simulink model "Copy_of_shake_table"  (Simulink 7.0)
settings: Solver=ode4  StartTime=0.0  StopTime=inf  FixedStep=0.001  RelTol=1e-3
undefined symbols (not defined in the file or in its folder): Den, Num, q
libraries: simulink x11, dsparch4 x5, xpclib x1
settings Model: Creator=Administrator  LastModifiedBy=msi  SimulationMode=external  BufferReuse=off
settings OptimizationCC: BlockReduction=off  OptimizeBlockIOStorage=off  BufferReuse=off  ExpressionFolding=off  LocalBlockOutputs=off
settings DebuggingCC: SaveWithParameterizedLinksMsg=none  SignalResolutionControl=TryResolveAllWithWarning
settings RTWCC: SystemTargetFile=xpctarget.tlc  TemplateMakefile=xpc_default_tmf  Description=xPC Target  ProcessScript=xpctarget_make_rtw_hook
settings xpcTargetCC: TargetFcnLib=ansi_tfl_tmw.mat  GenFloatMathFcnCalls=ANSI_C  CompOptLevelCompliant=off  PortableWordSizes=off  RL32LogBufSizeModifier=10000000

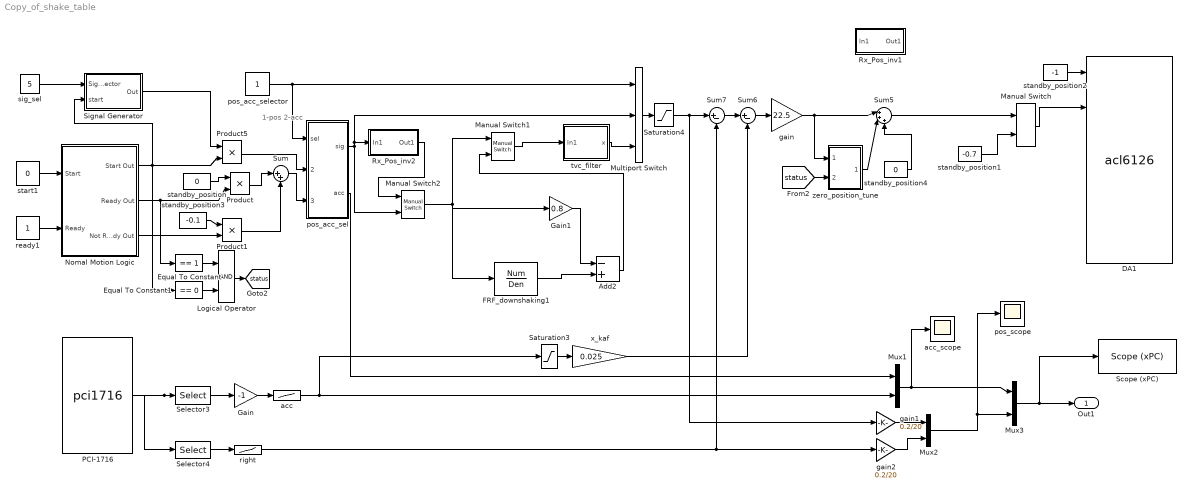
== system Copy_of_shake_table ==
  note: 1-pos
      | 2-acc
  Add2 : Sum  Inputs=-+  OutDataType=fixdt(1, 16)  OutScaling=2^-10
  DA1 : S-Function  FunctionName=acl6126  Parameters=convBaseAddr,Range,[SampleTime SampleOffset]  mask(ACL-6126){sBaseAddr=0x2C0, Ranges=-10, sample=0.001}
      mask prompts: sBaseAddr "Base Address:"; sample "Sample Time:"
      mask help:
      | ACL-6126
      | HIT
      | Analog Output
      mask init:
      | convBaseAddr = 512;Range=10;SampleTime = 0.001; SampleOffset = 0;
      | sampleLength = length (sample);
      | if (sampleLength == 2)
      |   SampleTime = sample(1);
      |   SampleOffset = sample(2);
      | else
      |   SampleTime = sample(1);
      |   SampleOffset = 0;
      | end
      | 
      | sBaseAddr(find(sBaseAddr=='''')) = [];
      | index = findstr(lower(sBaseAddr),'0x');
      | if ~isempty(index) & index==1
      |   BaseAddr = sBaseAddr(3:end);
      |   baLength = length (BaseAddr);
      |   baseStringMember = [abs('0'):abs('9'),abs('a'):abs('f'),abs('A'):abs('F')];
      |   for i = 1:baLength
      |  %   if ~ismember(BaseAddr(i),baseStringMember)
      |  %     error ('Invalid character in hexadecimal string');
      |  %   end
      |   end
      |   convBaseAddr = hex2dec(BaseAddr);
      | else
      |   convBaseAddr = str2num(BaseAddr);
      |   end
      |  Range=Ranges;
      mask Help: helpview([docroot '/toolbox/xpc/pt_io_block_reference.html#xpcioref'])
      mask Display:
      | disp('ACL-6126\ncumt\nAnalog Output');
      | port_label('input',1 , '1');
      | port_label('input',2 , '2');
      | port_label('input',3 , '3');
      | port_label('input',4 , '4');
      | port_label('input',5, '5');
      | port_label('input',6 , '6');
  Equal To Constant : simulink/Logic and Bit Operations/Compare To Constant  SystemSampleTime=-1  relop===  const=1  LogicOutDataTypeMode=uint8  ZeroCross=off
  Equal To Constant1 : simulink/Logic and Bit Operations/Compare To Constant  SystemSampleTime=-1  relop===  const=0  LogicOutDataTypeMode=uint8  ZeroCross=off
  FRF_downshaking1 : DiscreteTransferFcn  Numerator=Num  Denominator=Den  SampleTime=0.001
  Gain : Gain  Gain=-1  ParameterDataType=sfix(16)  ParameterScaling=2^0  OutDataType=sfix(16)  OutScaling=2^0  SaturateOnIntegerOverflow=on
  Gain1 : Gain  Gain=0.8  ParameterDataType=fixdt(1, 16)  ParameterScaling=2^0  OutDataType=fixdt(1, 16)  OutScaling=2^0
  Logical Operator : Logic  AllPortsSameDT=off
  Manual Switch : simulink/Signal Routing/Manual Switch  SystemSampleTime=-1  sw=1  action=0  varsize=off
  Manual Switch1 : simulink/Signal Routing/Manual Switch  SystemSampleTime=-1  sw=1  action=0  varsize=off
  Manual Switch2 : simulink/Signal Routing/Manual Switch  SystemSampleTime=-1  sw=0  action=0  varsize=off
  Multiport Switch : MultiPortSwitch  Inputs=2  SaturateOnIntegerOverflow=on
  Mux1 : Mux  Inputs=2
  Mux2 : Mux  Inputs=2
  Mux3 : Mux  Inputs=2
  Nomal Motion Logic : Subsystem  AncestorBlock=control_logic_lib/Control Logic(Stateflow Chart)
  PCI-1716 : S-Function  FunctionName=pci1716  Parameters=[SampleTime SampleOffset], SLOT  mask(hitad3){Sample=0.001, SLOT=-1}
      mask prompts: Sample "Sample Time:"
      mask help:
      | PCi1716
      | A/D Card
      | Developed by ZhaoJinsong
      | 2012.06.02
      mask init:
      | SampleTime = 0.001; SampleOffset=0;
      mask Help: helpview([docroot '/toolbox/xpc/pt_io_block_reference.html#xpcioref'])
      mask Display:
      | disp('PCI1716  ');
      | 
      | port_label('output',1 , 'OUT');
  Product : Product  OutDataType=sfix(16)  OutScaling=2^0  SaturateOnIntegerOverflow=on
  Product1 : Product  OutDataType=sfix(16)  OutScaling=2^0  SaturateOnIntegerOverflow=on
  Product5 : Product  OutDataType=sfix(16)  OutScaling=2^0  SaturateOnIntegerOverflow=on
  Rx_Pos_inv1 : Subsystem
  Rx_Pos_inv2 : Subsystem
  Saturation3 : Saturate  UpperLimit=2  LowerLimit=-2
  Saturation4 : Saturate  UpperLimit=10  LowerLimit=-10
  "Scope (xPC) " : xpclib/Misc./Scope (xPC)   SystemSampleTime=-1  scopeno=2  scopetype=Host  autostart=on  viewmode=Graphical redraw  formatstr='%15.6f'  grid=on  ylimits=[0,0]  nosamples=500  noprepostsamples=0  interleave=1  triggermode=FreeRun  triggersignal=1  triggerlevel=0.0  triggerslope=Either  triggerscope=1  triggersample=0  filename=data.dat  mode=Lazy  writesize=512  autorestart=off
  Selector3 : Selector  IndexOptions=Index vector (dialog)  Indices=[5]  OutputSizes=1
  Selector4 : Selector  IndexOptions=Index vector (dialog)  Indices=[3]  OutputSizes=1
  Signal Generator : Subsystem  TreatAsAtomicUnit=on
  Sum : Sum  Inputs=|++  OutDataType=sfix(16)  OutScaling=2^0  SaturateOnIntegerOverflow=on
  Sum5 : Sum  Inputs=|+++  OutDataType=sfix(16)  OutScaling=2^0  SaturateOnIntegerOverflow=on
  Sum6 : Sum  Inputs=|+-  OutDataType=sfix(16)  OutScaling=2^0  SaturateOnIntegerOverflow=on
  Sum7 : Sum  Inputs=|+-  OutDataType=sfix(16)  OutScaling=2^0  SaturateOnIntegerOverflow=on
  acc : Lookup  InputValues=[0.03 4.87]  Table=[0 1]  OutDataType=sfix(16)  OutScaling=2^0  SaturateOnIntegerOverflow=on
  acc_scope : Scope
      settings: TickLabels=on  TimeRange=1  YMin=-0.15  YMax=0.175
  gain : Gain  Gain=22.5  ParameterDataType=sfix(16)  ParameterScaling=2^0  OutDataType=sfix(16)  OutScaling=2^0  SaturateOnIntegerOverflow=on
  gain1 : Gain  Gain=0.2/20  ParameterDataType=sfix(16)  ParameterScaling=2^0  OutDataType=sfix(16)  OutScaling=2^0  SaturateOnIntegerOverflow=on
  gain2 : Gain  Gain=0.2/20  ParameterDataType=sfix(16)  ParameterScaling=2^0  OutDataType=sfix(16)  OutScaling=2^0  SaturateOnIntegerOverflow=on
  pos_acc_sel : Subsystem
  pos_acc_selector : Constant  OutDataType=sfix(16)  OutScaling=2^0
      settings: OpenFcn=|
      | if get_param(gcb,'value')=='1',
      | set_param(gcb,'value','2');
      | else
      | set_param(gcb,'value','1');end
  pos_scope : Scope
      settings: TickLabels=on  TimeRange=1  YMin=-0.00016  YMax=3e-005
  ready1 : Constant  OutDataType=sfix(16)  OutScaling=2^0
      settings: OpenFcn=|
      | if get_param(gcb,'value')=='1',
      | set_param(gcb,'value','0');
      | else
      | set_param(gcb,'value','1');end
  right : Lookup  InputValues=[2.007 9.834]  Table=[-10 10]  OutDataType=sfix(16)  OutScaling=2^0  SaturateOnIntegerOverflow=on
  sig_sel : Constant  Value=5  OutDataType=sfix(16)  OutScaling=2^0
  standby_position : Constant  Value=0  OutDataType=sfix(16)  OutScaling=2^0
  standby_position1 : Constant  Value=-0.7  OutDataType=sfix(16)  OutScaling=2^0
  standby_position2 : Constant  Value=-1  OutDataType=sfix(16)  OutScaling=2^0
  standby_position3 : Constant  Value=-0.1  OutDataType=sfix(16)  OutScaling=2^0
  standby_position4 : Constant  Value=0  OutDataType=sfix(16)  OutScaling=2^0
  start1 : Constant  Value=0  OutDataType=sfix(16)  OutScaling=2^0
      settings: OpenFcn=|
      | if get_param(gcb,'value')=='1',
      | set_param(gcb,'value','0');
      | else
      | set_param(gcb,'value','1');end
  tvc_filter : Subsystem
      mask Display: disp('Reference\nModule')
  x_kaf : Gain  Gain=0.025  ParameterDataType=sfix(16)  ParameterScaling=2^0  OutDataType=sfix(16)  OutScaling=2^0  SaturateOnIntegerOverflow=on
  zero_position_tune : Subsystem
  Out1 : Outport  OutDataType=sfix(16)  OutScaling=2^0
  tag scope: status=global
  wires:
  ready1/1 -> Nomal Motion Logic/2(Ready)
  start1/1 -> Nomal Motion Logic/1(Start)
  Nomal Motion Logic/2(Ready Out) -> Equal To Constant/1, Product/2
  standby_position/1 -> Product/1
  Product/1 -> Sum/1
  Sum/1 -> pos_acc_sel/3(ini_pos)
  Nomal Motion Logic/1(Start Out) -> Equal To Constant1/1, Product5/2, Signal Generator/2(start)
  Product5/1 -> pos_acc_sel/2(sig_in)
  Equal To Constant/1 -> Logical Operator/1
  Equal To Constant1/1 -> Logical Operator/2
  Logical Operator/1 -> [status]
  pos_acc_selector/1 -> Multiport Switch/1, pos_acc_sel/1(sel)
  Multiport Switch/1 -> Saturation4/1
  Saturation4/1 -> Sum7/1, gain1/1
  gain/1 -> Sum5/1, zero_position_tune/1(error_in)
  [status] -> zero_position_tune/2(status)
  zero_position_tune/1(Out) -> Sum5/2
  Sum5/1 -> Manual Switch/1
  acc/1 -> Mux1/2, Saturation3/1
  Saturation3/1 -> x_kaf/1
  x_kaf/1 -> Sum6/2
  Sum7/1 -> Sum6/1
  Sum6/1 -> gain/1
  Manual Switch/1 -> DA1/2
  gain1/1 -> Mux2/1
  PCI-1716/1 -> Selector3/1, Selector4/1
  Selector3/1 -> Gain/1
  Selector4/1 -> right/1
  Gain/1 -> acc/1
  gain2/1 -> Mux2/2
  standby_position2/1 -> DA1/1
  Mux1/1 -> Mux3/1, acc_scope/1
  Nomal Motion Logic/3(Not Ready Out) -> Product1/2
  standby_position3/1 -> Product1/1
  Mux3/1 -> "Scope (xPC) "/1, Out1/1
  Product1/1 -> Sum/2
  right/1 -> gain2/1, Sum7/2
  Mux2/1 -> Mux3/2, pos_scope/1
  standby_position1/1 -> Manual Switch/2
  sig_sel/1 -> Signal Generator/1(Signal Selector)
  Signal Generator/1(Out) -> Product5/1
  pos_acc_sel/2(acc) -> Mux1/1
  tvc_filter/1(x) -> Multiport Switch/3
  pos_acc_sel/1(sig) -> Multiport Switch/2, Rx_Pos_inv2/1(In1), Manual Switch2/2
  standby_position4/1 -> Sum5/3
  Manual Switch1/1 -> tvc_filter/1(In1)
  Gain1/1 -> Add2/1
  Add2/1 -> Manual Switch1/2
  FRF_downshaking1/1 -> Add2/2
  Manual Switch2/1 -> FRF_downshaking1/1, Manual Switch1/1, Gain1/1
  Rx_Pos_inv2/1(Out1) -> Manual Switch2/1

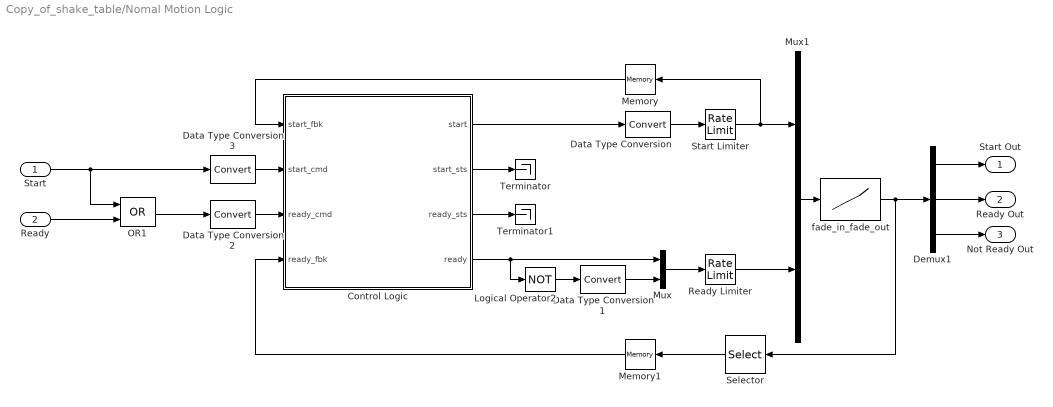
== system Copy_of_shake_table/Nomal Motion Logic ==
  Start : Inport  OutDataType=sfix(16)  OutScaling=2^0
  Ready : Inport  Port=2  OutDataType=sfix(16)  OutScaling=2^0
  Control Logic : Stateflow chart
  Data Type Conversion{,1..3} (4 alike) : DataTypeConversion  OutDataTypeMode=double  OutDataType=sfix(16)  OutScaling=2^0  SaturateOnIntegerOverflow=on  RndMeth=Zero
  Demux1 : Demux  Outputs=3
  Logical Operator2 : Logic  Operator=NOT  Inputs=3  AllPortsSameDT=off
  Memory : Memory  Orientation=left
  Memory1 : Memory  Orientation=left
  Mux : Mux  Inputs=2
  Mux1 : Mux  Inputs=2
  OR1 : Logic  Operator=OR  AllPortsSameDT=off
  Ready Limiter : RateLimiter  RisingSlewLimit=1/5  FallingSlewLimit=-1/5
  Selector : Selector  Orientation=left  InputPortWidth=3  IndexOptions=Index vector (dialog)  Indices=[2]  OutputSizes=1
  Start Limiter : RateLimiter  RisingSlewLimit=1/3  FallingSlewLimit=-1/3
  Terminator : Terminator
  Terminator1 : Terminator
  fade_in_fade_out : Lookup  InputValues=[0:0.001:1]  Table=(sin(([0:0.001:1]*2-1)*pi/2)+1)/2  OutDataType=sfix(16)  OutScaling=2^0  SaturateOnIntegerOverflow=on
  Start Out : Outport  OutDataType=sfix(16)  OutScaling=2^0
  Ready Out : Outport  Port=2  OutDataType=sfix(16)  OutScaling=2^0
  Not Ready Out : Outport  Port=3  OutDataType=sfix(16)  OutScaling=2^0
  wires:
  Ready/1 -> OR1/2
  Start/1 -> OR1/1, Data Type Conversion3/1
  Control Logic/3(ready_sts) -> Terminator1/1
  Control Logic/2(start_sts) -> Terminator/1
  OR1/1 -> Data Type Conversion2/1
  Data Type Conversion3/1 -> Control Logic/2(start_cmd)
  Demux1/3 -> Not Ready Out/1
  Demux1/1 -> Start Out/1
  Demux1/2 -> Ready Out/1
  Data Type Conversion/1 -> Start Limiter/1
  Start Limiter/1 -> Mux1/1, Memory/1
  Control Logic/1(start) -> Data Type Conversion/1
  Control Logic/4(ready) -> Logical Operator2/1, Mux/1
  Logical Operator2/1 -> Data Type Conversion1/1
  Mux/1 -> Ready Limiter/1
  Ready Limiter/1 -> Mux1/2
  Mux1/1 -> fade_in_fade_out/1
  fade_in_fade_out/1 -> Selector/1, Demux1/1
  Memory/1 -> Control Logic/1(start_fbk)
  Memory1/1 -> Control Logic/4(ready_fbk)
  Data Type Conversion1/1 -> Mux/2
  Data Type Conversion2/1 -> Control Logic/3(ready_cmd)
  Selector/1 -> Memory1/1

== system Copy_of_shake_table/Rx_Pos_inv1 ==
  In1 : Inport  OutDataType=sfix(16)  OutScaling=2^0
  Discrete Transfer Fcn1 : DiscreteTransferFcn  Numerator=[1 -0.2361]  Denominator=[1 0.3425]  SampleTime=0.001
  Discrete Transfer Fcn2 : DiscreteTransferFcn  Numerator=[1 -1.404 0.4961]  Denominator=[1 -1.59 0.7902]  SampleTime=0.001
  Discrete Transfer Fcn3 : DiscreteTransferFcn  Numerator=[1 -1.808 0.9141]  Denominator=[1.666 -2.372 1]  SampleTime=0.001
  Discrete Transfer Fcn4 : DiscreteTransferFcn  Numerator=[1 1.076 0.8841]  Denominator=[1 -1.303 0.8939]  SampleTime=0.001
  Discrete Transfer Fcn6 : DiscreteTransferFcn  Numerator=[1 -0.06054 0.6042]  Denominator=[1 0.5145 0.7374]  SampleTime=0.001
  Gain : Gain  Gain=1/0.31645  ParameterDataType=sfix(16)  ParameterScaling=2^0  OutDataType=sfix(16)  OutScaling=2^0
  Gain1 : Gain  ParameterDataType=sfix(16)  ParameterScaling=2^0  OutDataType=sfix(16)  OutScaling=2^0
  Out1 : Outport  OutDataType=sfix(16)  OutScaling=2^0
  wires:
  Discrete Transfer Fcn1/1 -> Discrete Transfer Fcn2/1
  Discrete Transfer Fcn2/1 -> Discrete Transfer Fcn3/1
  Discrete Transfer Fcn3/1 -> Discrete Transfer Fcn4/1
  Discrete Transfer Fcn4/1 -> Discrete Transfer Fcn6/1
  Discrete Transfer Fcn6/1 -> Gain/1
  In1/1 -> Discrete Transfer Fcn1/1
  Gain/1 -> Gain1/1
  Gain1/1 -> Out1/1

== system Copy_of_shake_table/Rx_Pos_inv2 ==
  In1 : Inport  OutDataType=sfix(16)  OutScaling=2^0
  Discrete Transfer Fcn1 : DiscreteTransferFcn  Numerator=[1 0.2074]  Denominator=[1.002 -1]  SampleTime=0.001
  Discrete Transfer Fcn2 : DiscreteTransferFcn  Numerator=[1 -1]  Denominator=[1 -0.8636]  SampleTime=0.001
  Discrete Transfer Fcn3 : DiscreteTransferFcn  Numerator=[1 -1.866 0.8774]  Denominator=[1 -1.762 0.9049]  SampleTime=0.001
  Discrete Transfer Fcn4 : DiscreteTransferFcn  Numerator=[1 -1.828 0.9273]  Denominator=[1 -0.4559 0.3103]  SampleTime=0.001
  Discrete Transfer Fcn5 : DiscreteTransferFcn  Numerator=[1 -1.652 0.9951]  Denominator=[1.96 -2.518 1]  SampleTime=0.001
  Discrete Transfer Fcn6 : DiscreteTransferFcn  Numerator=[1 -1.779 0.9237]  Denominator=[1 -1.656 0.9996]  SampleTime=0.001
  Gain : Gain  Gain=1/0.02213  ParameterDataType=sfix(16)  ParameterScaling=2^0  OutDataType=sfix(16)  OutScaling=2^0
  Gain1 : Gain  ParameterDataType=sfix(16)  ParameterScaling=2^0  OutDataType=sfix(16)  OutScaling=2^0
  Out1 : Outport  OutDataType=sfix(16)  OutScaling=2^0
  wires:
  Discrete Transfer Fcn1/1 -> Discrete Transfer Fcn2/1
  Discrete Transfer Fcn2/1 -> Discrete Transfer Fcn3/1
  Discrete Transfer Fcn3/1 -> Discrete Transfer Fcn4/1
  Discrete Transfer Fcn4/1 -> Discrete Transfer Fcn6/1
  Discrete Transfer Fcn6/1 -> Discrete Transfer Fcn5/1
  In1/1 -> Discrete Transfer Fcn1/1
  Gain/1 -> Gain1/1
  Gain1/1 -> Out1/1
  Discrete Transfer Fcn5/1 -> Gain/1

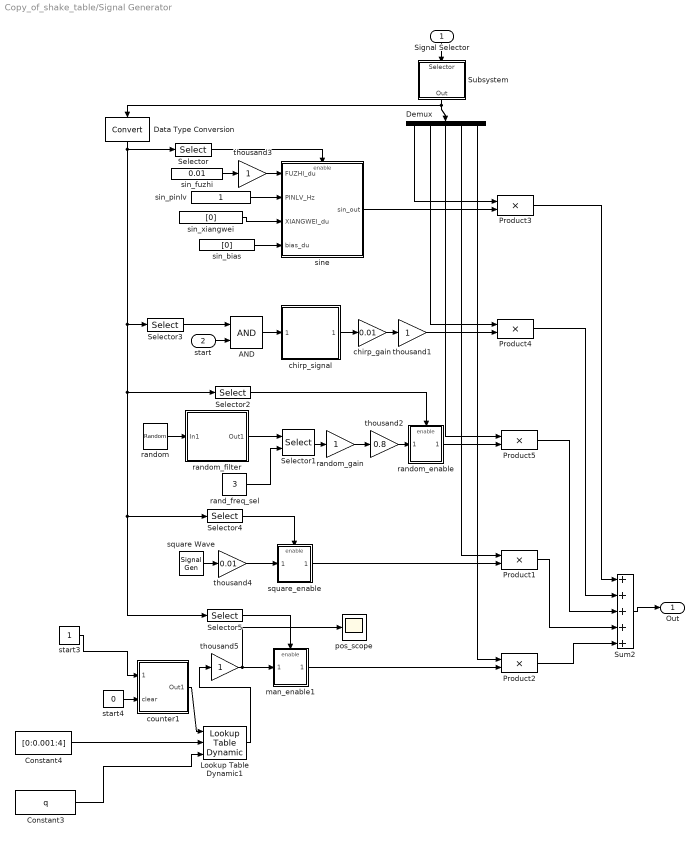
== system Copy_of_shake_table/Signal Generator ==
  Signal Selector : Inport  Orientation=down  OutDataType=sfix(16)  OutScaling=2^0
  start : Inport  Port=2  OutDataType=sfix(16)  OutScaling=2^0
  AND : Logic  AllPortsSameDT=off  OutDataTypeMode=Specify via dialog
  Constant3 : Constant  Value=q  OutDataType=sfix(16)  OutScaling=2^0
  Constant4 : Constant  Value=[0:0.001:4]  OutDataType=sfix(16)  OutScaling=2^0
  Data Type Conversion : DataTypeConversion  Orientation=down  OutDataTypeMode=boolean  OutDataType=sfix(16)  OutScaling=2^0  SaturateOnIntegerOverflow=on  RndMeth=Zero
  Demux : Demux  Orientation=down  Outputs=5
  Lookup Table Dynamic1 : simulink/Lookup Tables/Lookup Table Dynamic  LookUpMeth=Interpolation-Use End Values  OutDataTypeStr=float('double')  OutputDataTypeScalingMode=Specify via dialog  OutDataType=float('double')  OutScaling=2^-10  DoSatur=off
  Product{1..5} (5 alike) : Product  OutDataType=sfix(16)  OutScaling=2^0  SaturateOnIntegerOverflow=on
  Selector : Selector  InputPortWidth=5  IndexOptions=Index vector (dialog)  Indices=1  OutputSizes=1
  Selector1 : Selector  InputPortWidth=5  IndexOptions=Index vector (port)  Indices=[1 3]  OutputSizes=1
  Selector2 : Selector  InputPortWidth=5  IndexOptions=Index vector (dialog)  Indices=3  OutputSizes=1
  Selector3 : Selector  InputPortWidth=5  IndexOptions=Index vector (dialog)  Indices=2  OutputSizes=1
  Selector4 : Selector  InputPortWidth=5  IndexOptions=Index vector (dialog)  Indices=4  OutputSizes=1
  Selector5 : Selector  InputPortWidth=5  IndexOptions=Index vector (dialog)  Indices=5  OutputSizes=1
  Subsystem : Subsystem  Orientation=down  mask{itnum=5}
      mask prompts: itnum "Signals Number"
  Sum2 : Sum  Inputs=+++++  OutDataType=sfix(16)  OutScaling=2^0  SaturateOnIntegerOverflow=on
  chirp_gain : Gain  Gain=0.01  ParameterDataType=sfix(16)  ParameterScaling=2^0  OutDataType=sfix(16)  OutScaling=2^0  SaturateOnIntegerOverflow=on
  chirp_signal : Subsystem
  counter1 : Subsystem
  man_enable1 : Subsystem  TreatAsAtomicUnit=on
  pos_scope : Scope
      settings: TickLabels=on  TimeRange=1  YMin=-4.25  YMax=0.75  SaveName=ScopeData2
  rand_freq_sel : Constant  Value=3  OutDataType=sfix(16)  OutScaling=2^0
  random : UniformRandomNumber  SampleTime=0
  random_enable : Subsystem  TreatAsAtomicUnit=on
  random_filter : Subsystem
  random_gain : Gain  ParameterDataType=sfix(16)  ParameterScaling=2^0  OutDataType=sfix(16)  OutScaling=2^0  SaturateOnIntegerOverflow=on
  sin_bias : Constant  Value=[0]  OutDataType=sfix(16)  OutScaling=2^0
  sin_fuzhi : Constant  Value=0.01  OutDataType=sfix(16)  OutScaling=2^0
  sin_pinlv : Constant  OutDataType=sfix(16)  OutScaling=2^0
  sin_xiangwei : Constant  Value=[0]  OutDataType=sfix(16)  OutScaling=2^0
  sine : Subsystem
  square Wave : SignalGenerator  WaveForm=square  Frequency=0.1
  square_enable : Subsystem  TreatAsAtomicUnit=on
  start3 : Constant  OutDataType=sfix(16)  OutScaling=2^0
      settings: OpenFcn=|
      | if strcmp(get_param(gcb,'Value'),'1')
      | set_param(gcb,'Value','0');
      | else
      | set_param(gcb,'Value','1');
      | end;
  start4 : Constant  Value=0  OutDataType=sfix(16)  OutScaling=2^0
      settings: OpenFcn=|
      | if strcmp(get_param(gcb,'Value'),'1')
      | set_param(gcb,'Value','0');
      | else
      | set_param(gcb,'Value','1');
      | end;
  thousand1 : Gain  ParameterDataType=sfix(16)  ParameterScaling=2^0  OutDataType=sfix(16)  OutScaling=2^0  SaturateOnIntegerOverflow=on
  thousand2 : Gain  Gain=0.8  ParameterDataType=sfix(16)  ParameterScaling=2^0  OutDataType=sfix(16)  OutScaling=2^0  SaturateOnIntegerOverflow=on
  thousand3 : Gain  ParameterDataType=sfix(16)  ParameterScaling=2^0  OutDataType=sfix(16)  OutScaling=2^0  SaturateOnIntegerOverflow=on
  thousand4 : Gain  Gain=0.01  ParameterDataType=sfix(16)  ParameterScaling=2^0  OutDataType=sfix(16)  OutScaling=2^0  SaturateOnIntegerOverflow=on
  thousand5 : Gain  ParameterDataType=sfix(16)  ParameterScaling=2^0  OutDataType=sfix(16)  OutScaling=2^0  SaturateOnIntegerOverflow=on
  Out : Outport  OutDataType=sfix(16)  OutScaling=2^0
  wires:
  thousand1/1 -> Product4/2
  chirp_signal/1(chirp_signal) -> chirp_gain/1
  AND/1 -> chirp_signal/1(enable)
  chirp_gain/1 -> thousand1/1
  start/1 -> AND/2
  Selector3/1 -> AND/1
  thousand4/1 -> square_enable/1(In1)
  thousand3/1 -> sine/1(FUZHI_du)
  square_enable/1(Out1) -> Product1/2
  Selector4/1 -> square_enable/Enable
  square Wave/1 -> thousand4/1
  random_gain/1 -> thousand2/1
  thousand2/1 -> random_enable/1(In1)
  Selector1/1 -> random_gain/1
  Signal Selector/1 -> Subsystem/1(Selector)
  Product4/1 -> Sum2/2
  Product3/1 -> Sum2/1
  Product5/1 -> Sum2/3
  Sum2/1 -> Out/1
  Subsystem/1(Out) -> Demux/1, Data Type Conversion/1
  sin_bias/1 -> sine/4(bias_du)
  sin_xiangwei/1 -> sine/3(XIANGWEI_du)
  sin_pinlv/1 -> sine/2(PINLV_Hz)
  sin_fuzhi/1 -> thousand3/1
  Selector/1 -> sine/Enable
  Data Type Conversion/1 -> Selector/1, Selector3/1, Selector2/1, Selector4/1, Selector5/1
  random/1 -> random_filter/1(In1)
  random_filter/1(Out1) -> Selector1/1
  rand_freq_sel/1 -> Selector1/2
  Selector2/1 -> random_enable/Enable
  Demux/1 -> Product3/1
  sine/1(sin_out) -> Product3/2
  Demux/2 -> Product4/1
  Demux/3 -> Product5/1
  random_enable/1(Out1) -> Product5/2
  Demux/4 -> Product1/1
  Product1/1 -> Sum2/4
  Selector5/1 -> man_enable1/Enable
  man_enable1/1(Out1) -> Product2/2
  Demux/5 -> Product2/1
  Product2/1 -> Sum2/5
  thousand5/1 -> man_enable1/1(In1), pos_scope/1
  Constant4/1 -> Lookup Table Dynamic1/2
  Constant3/1 -> Lookup Table Dynamic1/3
  start3/1 -> counter1/1(codition)
  start4/1 -> counter1/2(clear)
  counter1/1(Out1) -> Lookup Table Dynamic1/1
  Lookup Table Dynamic1/1 -> thousand5/1

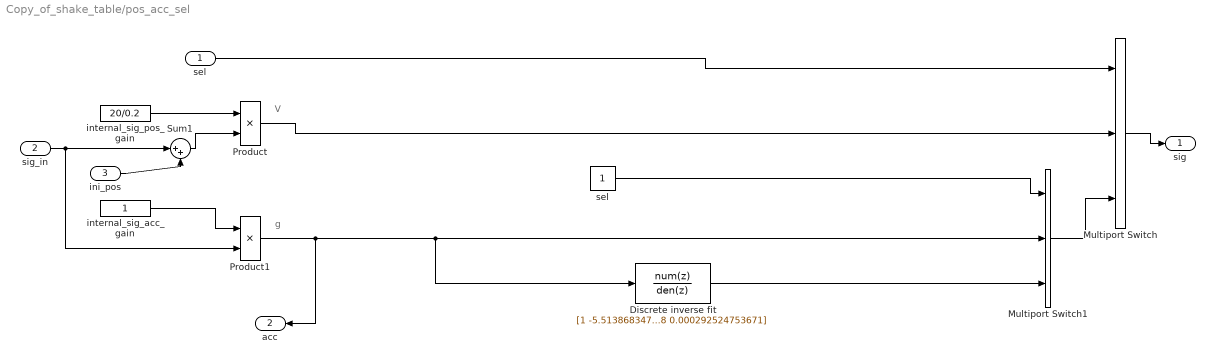
== system Copy_of_shake_table/pos_acc_sel ==
  note: g
  note: V
  sel : Inport  OutDataType=sfix(16)  OutScaling=2^0
  sig_in : Inport  Port=2  OutDataType=sfix(16)  OutScaling=2^0
  ini_pos : Inport  Port=3  OutDataType=sfix(16)  OutScaling=2^0
  Discrete inverse fit : DiscreteTransferFcn  Numerator=[1 -5.513868347662695 12.88491366007906 -16.323990002559352 11.821537968329908 -4.639485908156727 0.77101716333547]  Denominator=[0.013392688630559 -0.043519228995354 0.057088791124972 -0.038794303856191 0.015270049598488 -0.003637012524308 0.000292524753671]  SampleTime=0.001
  Multiport Switch : MultiPortSwitch  Inputs=2  SaturateOnIntegerOverflow=on
  Multiport Switch1 : MultiPortSwitch  Inputs=2  SaturateOnIntegerOverflow=on
  Product : Product  OutDataType=sfix(16)  OutScaling=2^0  SaturateOnIntegerOverflow=on
  Product1 : Product  OutDataType=sfix(16)  OutScaling=2^0  SaturateOnIntegerOverflow=on
  Sum1 : Sum  Inputs=|++  OutDataType=sfix(16)  OutScaling=2^0  SaturateOnIntegerOverflow=on
  internal_sig_acc_gain : Constant  OutDataType=sfix(16)  OutScaling=2^0
  internal_sig_pos_gain : Constant  Value=20/0.2  OutDataType=sfix(16)  OutScaling=2^0
  "sel " : Constant  OutDataType=sfix(16)  OutScaling=2^0
  sig : Outport  OutDataType=sfix(16)  OutScaling=2^0
  acc : Outport  Orientation=left  Port=2  OutDataType=sfix(16)  OutScaling=2^0
  wires:
  internal_sig_acc_gain/1 -> Product1/1
  Product1/1 -> Discrete inverse fit/1, Multiport Switch1/2, acc/1
  internal_sig_pos_gain/1 -> Product/1
  Product/1 -> Multiport Switch/2
  Sum1/1 -> Product/2
  ini_pos/1 -> Sum1/2
  Multiport Switch/1 -> sig/1
  sel/1 -> Multiport Switch/1
  sig_in/1 -> Product1/2, Sum1/1
  Discrete inverse fit/1 -> Multiport Switch1/3
  "sel "/1 -> Multiport Switch1/1
  Multiport Switch1/1 -> Multiport Switch/3

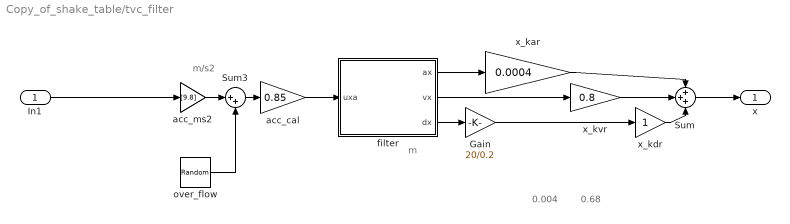
== system Copy_of_shake_table/tvc_filter ==
  note: m/s2
  note: m
  note: 0.004
  note: 0.68
  In1 : Inport  OutDataType=sfix(16)  OutScaling=2^0
  Gain : Gain  Gain=20/0.2  ParameterDataType=sfix(16)  ParameterScaling=2^0  OutDataType=sfix(16)  OutScaling=2^0  SaturateOnIntegerOverflow=on
  Sum : Sum  Inputs=+++  OutDataType=sfix(16)  OutScaling=2^0  SaturateOnIntegerOverflow=on
  Sum3 : Sum  Inputs=|++  OutDataType=sfix(16)  OutScaling=2^0  SaturateOnIntegerOverflow=on
  acc_cal : Gain  Gain=0.85  ParameterDataType=sfix(16)  ParameterScaling=2^0  OutDataType=sfix(16)  OutScaling=2^0  SaturateOnIntegerOverflow=on
  acc_ms2 : Gain  Gain=[9.8]  ParameterDataType=sfix(16)  ParameterScaling=2^0  OutDataType=sfix(16)  OutScaling=2^0  SaturateOnIntegerOverflow=on
  filter : Subsystem
      mask Display: disp('x_filter')
  over_flow : RandomNumber  Variance=1e-10  SampleTime=0
  x_kar : Gain  Gain=0.0004  ParameterDataType=sfix(16)  ParameterScaling=2^0  OutDataType=sfix(16)  OutScaling=2^0  SaturateOnIntegerOverflow=on
  x_kdr : Gain  ParameterDataType=sfix(16)  ParameterScaling=2^0  OutDataType=sfix(16)  OutScaling=2^0  SaturateOnIntegerOverflow=on
  x_kvr : Gain  Gain=0.8  ParameterDataType=sfix(16)  ParameterScaling=2^0  OutDataType=sfix(16)  OutScaling=2^0  SaturateOnIntegerOverflow=on
  x : Outport  OutDataType=sfix(16)  OutScaling=2^0
  wires:
  over_flow/1 -> Sum3/2
  In1/1 -> acc_ms2/1
  Sum3/1 -> acc_cal/1
  acc_ms2/1 -> Sum3/1
  acc_cal/1 -> filter/1(uxa)
  x_kdr/1 -> Sum/3
  x_kvr/1 -> Sum/2
  x_kar/1 -> Sum/1
  filter/1(ax) -> x_kar/1
  filter/2(vx) -> x_kvr/1
  filter/3(dx) -> Gain/1
  Sum/1 -> x/1
  Gain/1 -> x_kdr/1

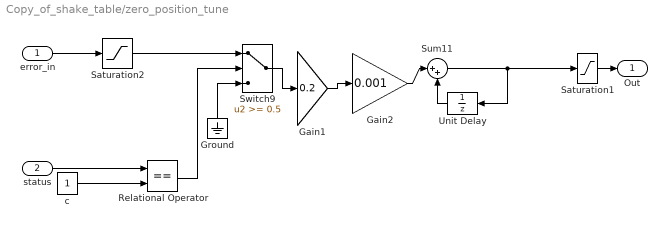
== system Copy_of_shake_table/zero_position_tune ==
  error_in : Inport  OutDataType=sfix(16)  OutScaling=2^0
  status : Inport  Port=2  OutDataType=sfix(16)  OutScaling=2^0
  Gain1 : Gain  Gain=0.2  ParameterDataType=sfix(16)  ParameterScaling=2^0  OutDataType=sfix(16)  OutScaling=2^0  SaturateOnIntegerOverflow=on
  Gain2 : Gain  Gain=0.001  ParameterDataType=sfix(16)  ParameterScaling=2^0  OutDataType=sfix(16)  OutScaling=2^0  SaturateOnIntegerOverflow=on
  Ground : Ground  Orientation=up
  Relational Operator : RelationalOperator  Operator===  InputSameDT=on
  Saturation1 : Saturate
  Saturation2 : Saturate  UpperLimit=0.1  LowerLimit=-0.1
  Sum11 : Sum  Inputs=|++  OutDataType=sfix(16)  OutScaling=2^0  SaturateOnIntegerOverflow=on  InputSameDT=on
  Switch9 : Switch  Threshold=0.5  SaturateOnIntegerOverflow=on  InputSameDT=on
  Unit Delay : UnitDelay  Orientation=left  X0=-0.03  SampleTime=0.001
  c : Constant  OutDataTypeMode=boolean  OutDataType=sfix(16)  OutScaling=2^0
  Out : Outport  OutDataType=sfix(16)  OutScaling=2^0
  wires:
  Saturation1/1 -> Out/1
  Gain1/1 -> Gain2/1
  status/1 -> Relational Operator/1
  error_in/1 -> Saturation2/1
  Relational Operator/1 -> Switch9/2
  c/1 -> Relational Operator/2
  Saturation2/1 -> Switch9/1
  Ground/1 -> Switch9/3
  Switch9/1 -> Gain1/1
  Sum11/1 -> Saturation1/1, Unit Delay/1
  Gain2/1 -> Sum11/1
  Unit Delay/1 -> Sum11/2

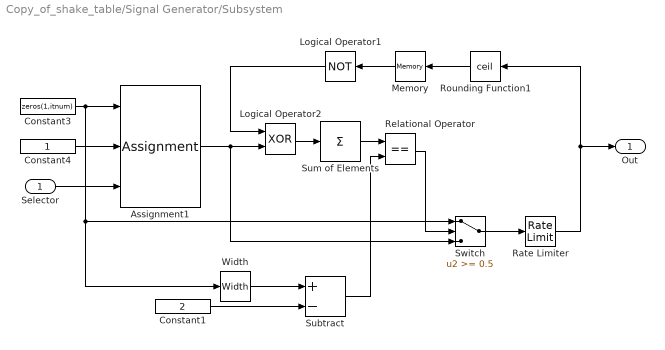
== system Copy_of_shake_table/Signal Generator/Subsystem ==
  Selector : Inport  OutDataType=sfix(16)  OutScaling=2^0
  Assignment1 : Assignment  IndexOptions=Index vector (port)  Indices=1  OutputSizes=[1]
  Constant1 : Constant  Value=2  OutDataType=sfix(16)  OutScaling=2^0
  Constant3 : Constant  Value=zeros(1,itnum)  OutDataType=sfix(16)  OutScaling=2^0
  Constant4 : Constant  OutDataType=sfix(16)  OutScaling=2^0
  Logical Operator1 : Logic  Orientation=left  Operator=NOT  AllPortsSameDT=off
  Logical Operator2 : Logic  Operator=XOR  AllPortsSameDT=off
  Memory : Memory  Orientation=left  InheritSampleTime=on
  Rate Limiter : RateLimiter
  Relational Operator : RelationalOperator  Operator===
  Rounding Function1 : Rounding  Orientation=left  Operator=ceil
  Subtract : Sum  Inputs=+-  OutDataTypeMode=double  OutDataType=sfix(16)  OutScaling=2^-10
  Sum of Elements : Sum  Inputs=+  OutDataTypeMode=double  OutDataType=sfix(16)  OutScaling=2^-10
  Switch : Switch  Threshold=0.5  SaturateOnIntegerOverflow=on
  Width : Width
  Out : Outport  OutDataType=sfix(16)  OutScaling=2^0
  wires:
  Constant3/1 -> Assignment1/1, Width/1, Switch/1
  Constant4/1 -> Assignment1/2
  Assignment1/1 -> Logical Operator2/2, Switch/3
  Rate Limiter/1 -> Rounding Function1/1, Out/1
  Rounding Function1/1 -> Memory/1
  Logical Operator1/1 -> Logical Operator2/1
  Switch/1 -> Rate Limiter/1
  Memory/1 -> Logical Operator1/1
  Selector/1 -> Assignment1/3
  Logical Operator2/1 -> Sum of Elements/1
  Width/1 -> Subtract/1
  Constant1/1 -> Subtract/2
  Sum of Elements/1 -> Relational Operator/1
  Subtract/1 -> Relational Operator/2
  Relational Operator/1 -> Switch/2

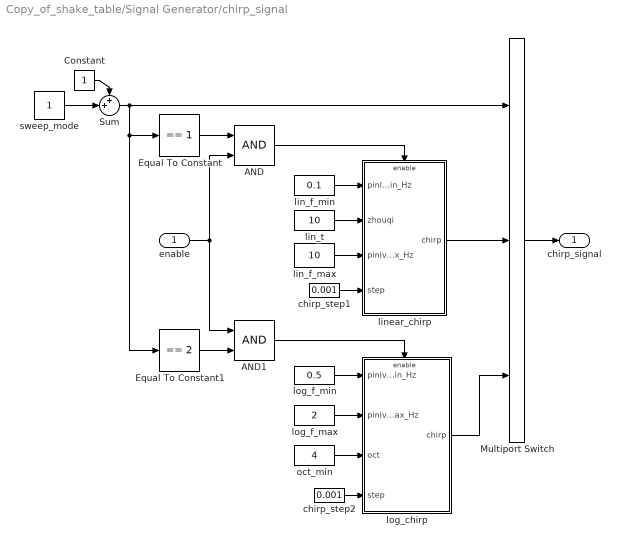
== system Copy_of_shake_table/Signal Generator/chirp_signal ==
  enable : Inport  OutDataType=sfix(16)  OutScaling=2^0
  AND : Logic  AllPortsSameDT=off  OutDataTypeMode=Specify via dialog
  AND1 : Logic  AllPortsSameDT=off  OutDataTypeMode=Specify via dialog
  Constant : Constant  OutDataType=sfix(16)  OutScaling=2^0
  Equal To Constant : simulink/Logic and Bit Operations/Compare To Constant  SystemSampleTime=-1  relop===  const=1  LogicOutDataTypeMode=uint8  ZeroCross=off
  Equal To Constant1 : simulink/Logic and Bit Operations/Compare To Constant  SystemSampleTime=-1  relop===  const=2  LogicOutDataTypeMode=uint8  ZeroCross=off
  Multiport Switch : MultiPortSwitch  Inputs=2  SaturateOnIntegerOverflow=on
  Sum : Sum  Inputs=++|  OutDataType=sfix(16)  OutScaling=2^0  SaturateOnIntegerOverflow=on
  chirp_step1 : Constant  Value=0.001  OutDataType=sfix(16)  OutScaling=2^0
  chirp_step2 : Constant  Value=0.001  OutDataType=sfix(16)  OutScaling=2^0
  lin_f_max : Constant  Value=10  OutDataType=sfix(16)  OutScaling=2^0
  lin_f_min : Constant  Value=0.1  OutDataType=sfix(16)  OutScaling=2^0
  lin_t : Constant  Value=10  OutDataType=sfix(16)  OutScaling=2^0
  linear_chirp : Subsystem
  log_chirp : Subsystem
  log_f_max : Constant  Value=2  OutDataType=sfix(16)  OutScaling=2^0
  log_f_min : Constant  Value=0.5  OutDataType=sfix(16)  OutScaling=2^0
  oct_min : Constant  Value=4  OutDataType=sfix(16)  OutScaling=2^0
  sweep_mode : Constant  OutDataType=sfix(16)  OutScaling=2^0
  chirp_signal : Outport  OutDataType=sfix(16)  OutScaling=2^0
  wires:
  AND/1 -> linear_chirp/Enable
  AND1/1 -> log_chirp/Enable
  enable/1 -> AND1/1, AND/2
  Equal To Constant1/1 -> AND1/2
  Equal To Constant/1 -> AND/1
  Sum/1 -> Equal To Constant1/1, Equal To Constant/1, Multiport Switch/1
  linear_chirp/1(chirp) -> Multiport Switch/2
  log_chirp/1(chirp) -> Multiport Switch/3
  Constant/1 -> Sum/1
  sweep_mode/1 -> Sum/2
  Multiport Switch/1 -> chirp_signal/1
  chirp_step2/1 -> log_chirp/4(step)
  chirp_step1/1 -> linear_chirp/4(step)
  lin_t/1 -> linear_chirp/2(zhouqi)
  lin_f_max/1 -> linear_chirp/3(pinlv_max_Hz)
  lin_f_min/1 -> linear_chirp/1(pinlv_min_Hz)
  oct_min/1 -> log_chirp/3(oct)
  log_f_max/1 -> log_chirp/2(pinlv_max_Hz)
  log_f_min/1 -> log_chirp/1(pinlv_min_Hz)

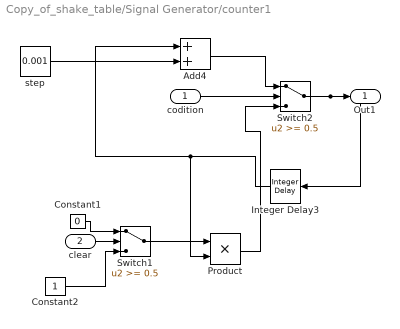
== system Copy_of_shake_table/Signal Generator/counter1 ==
  codition : Inport  OutDataType=sfix(16)  OutScaling=2^0
  clear : Inport  Port=2  OutDataType=sfix(16)  OutScaling=2^0
  Add4 : Sum  OutDataType=sfix(16)  OutScaling=2^-10
  Constant1 : Constant  Value=0  OutDataType=sfix(16)  OutScaling=2^0
  Constant2 : Constant  OutDataType=sfix(16)  OutScaling=2^0
  Integer Delay3 : simulink/Discrete/Integer Delay  Orientation=left  vinit=0.0  samptime=-1  NumDelays=1
  Product : Product  OutDataType=sfix(16)  OutScaling=2^0  RndMeth=Zero
  Switch1 : Switch  Threshold=0.5
  Switch2 : Switch  Threshold=0.5
  step : Constant  Value=0.001  OutDataType=sfix(16)  OutScaling=2^0
  Out1 : Outport  OutDataType=sfix(16)  OutScaling=2^0
  wires:
  Constant2/1 -> Switch1/3
  clear/1 -> Switch1/2
  codition/1 -> Switch2/2
  Product/1 -> Switch2/3
  Constant1/1 -> Switch1/1
  Switch1/1 -> Product/1
  step/1 -> Add4/2
  Integer Delay3/1 -> Product/2, Add4/1
  Switch2/1 -> Out1/1, Integer Delay3/1
  Add4/1 -> Switch2/1

== system Copy_of_shake_table/Signal Generator/man_enable1 ==
  In1 : Inport  OutDataType=sfix(16)  OutScaling=2^0
  Enable : EnablePort  StatesWhenEnabling=reset
  Out1 : Outport  OutDataType=sfix(16)  OutScaling=2^0
  wires:
  In1/1 -> Out1/1

== system Copy_of_shake_table/Signal Generator/random_enable ==
  In1 : Inport  OutDataType=sfix(16)  OutScaling=2^0
  Enable : EnablePort  StatesWhenEnabling=reset
  Out1 : Outport  OutDataType=sfix(16)  OutScaling=2^0
  wires:
  In1/1 -> Out1/1

== system Copy_of_shake_table/Signal Generator/random_filter ==
  In1 : Inport  OutDataType=sfix(16)  OutScaling=2^0
  1-10 : dsparch4/Analog Filter Design  method=Butterworth  filttype=Bandpass  N=8  Wlo=1*2*pi  Whi=10*2*pi  Rp=2  Rs=40
  2-100 : dsparch4/Analog Filter Design  method=Butterworth  filttype=Bandpass  N=8  Wlo=2*2*pi  Whi=100*2*pi  Rp=2  Rs=40
  2-200 : dsparch4/Analog Filter Design  method=Butterworth  filttype=Bandpass  N=8  Wlo=2*2*pi  Whi=200*2*pi  Rp=2  Rs=40
  2-45 : dsparch4/Analog Filter Design  method=Butterworth  filttype=Bandpass  N=8  Wlo=2*2*pi  Whi=45*2*pi  Rp=2  Rs=40
  4-20 : dsparch4/Analog Filter Design  method=Butterworth  filttype=Bandpass  N=8  Wlo=4*2*pi  Whi=20*2*pi  Rp=2  Rs=40
  Mux : Mux  Inputs=5
  Out1 : Outport  OutDataType=sfix(16)  OutScaling=2^0
  wires:
  In1/1 -> 2-200/1, 1-10/1, 2-100/1, 4-20/1, 2-45/1
  2-45/1 -> Mux/1
  4-20/1 -> Mux/2
  2-100/1 -> Mux/3
  1-10/1 -> Mux/4
  2-200/1 -> Mux/5
  Mux/1 -> Out1/1

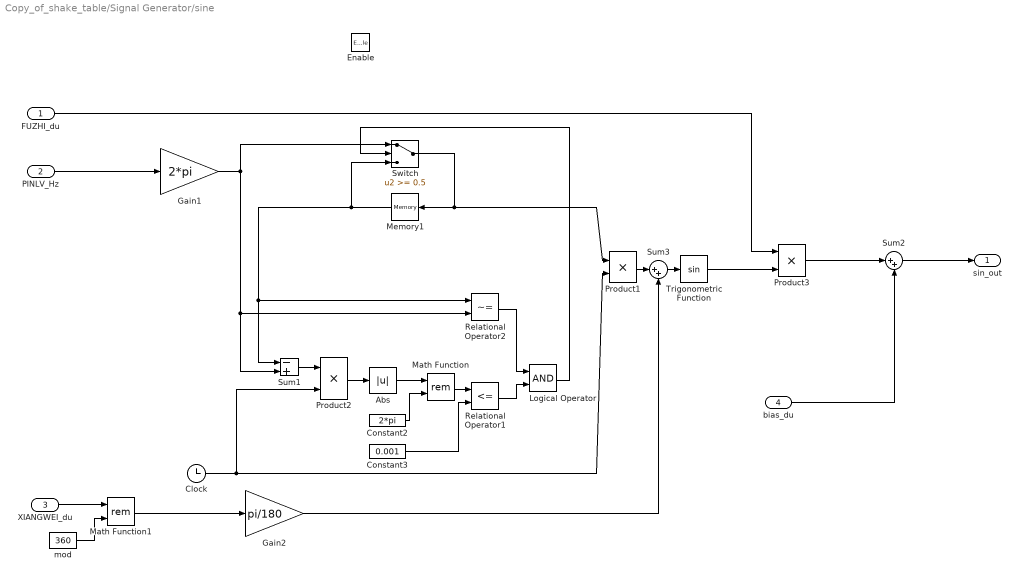
== system Copy_of_shake_table/Signal Generator/sine ==
  FUZHI_du : Inport  OutDataType=sfix(16)  OutScaling=2^0
  PINLV_Hz : Inport  Port=2  OutDataType=sfix(16)  OutScaling=2^0
  XIANGWEI_du : Inport  Port=3  OutDataType=sfix(16)  OutScaling=2^0
  bias_du : Inport  Port=4  OutDataType=sfix(16)  OutScaling=2^0
  Enable : EnablePort  StatesWhenEnabling=reset
  Abs : Abs  SaturateOnIntegerOverflow=on
  Clock : Clock
      settings: Decimation=10
  Constant2 : Constant  Value=2*pi  OutDataType=sfix(16)  OutScaling=2^0
  Constant3 : Constant  Value=0.001  OutDataType=sfix(16)  OutScaling=2^0
  Gain1 : Gain  Gain=2*pi  ParameterDataType=sfix(16)  ParameterScaling=2^0  OutDataType=sfix(16)  OutScaling=2^0  SaturateOnIntegerOverflow=on
  Gain2 : Gain  Gain=pi/180  ParameterDataType=sfix(16)  ParameterScaling=2^0  OutDataType=sfix(16)  OutScaling=2^0  SaturateOnIntegerOverflow=on
  Logical Operator : Logic  AllPortsSameDT=off
  Math Function : Math  Operator=rem  OutDataType=sfix(16)  OutScaling=2^0  SaturateOnIntegerOverflow=on
  Math Function1 : Math  Operator=rem  OutDataType=sfix(16)  OutScaling=2^0  SaturateOnIntegerOverflow=on
  Memory1 : Memory  Orientation=left  X0=[0]
  Product1 : Product  OutDataType=sfix(16)  OutScaling=2^0  SaturateOnIntegerOverflow=on
  Product2 : Product  OutDataType=sfix(16)  OutScaling=2^0  SaturateOnIntegerOverflow=on
  Product3 : Product  OutDataType=sfix(16)  OutScaling=2^0  SaturateOnIntegerOverflow=on
  Relational Operator1 : RelationalOperator  Operator=<=
  Relational Operator2 : RelationalOperator  Operator=~=
  Sum1 : Sum  Inputs=-+  OutDataType=sfix(16)  OutScaling=2^0  SaturateOnIntegerOverflow=on
  Sum2 : Sum  Inputs=|++  OutDataType=sfix(16)  OutScaling=2^0  SaturateOnIntegerOverflow=on
  Sum3 : Sum  Inputs=|++  OutDataType=sfix(16)  OutScaling=2^0  SaturateOnIntegerOverflow=on
  Switch : Switch  Threshold=0.5  SaturateOnIntegerOverflow=on
  Trigonometric Function : Trigonometry
  mod : Constant  Value=360  OutDataType=sfix(16)  OutScaling=2^0
  sin_out : Outport  OutDataType=sfix(16)  OutScaling=2^0
  wires:
  Product1/1 -> Sum3/1
  Clock/1 -> Product1/2, Product2/2
  Trigonometric Function/1 -> Product3/2
  Gain2/1 -> Sum3/2
  Sum3/1 -> Trigonometric Function/1
  FUZHI_du/1 -> Product3/1
  Product2/1 -> Abs/1
  Abs/1 -> Math Function/1
  Constant2/1 -> Math Function/2
  Math Function/1 -> Relational Operator1/1
  Constant3/1 -> Relational Operator1/2
  Switch/1 -> Memory1/1, Product1/1
  Gain1/1 -> Relational Operator2/2, Sum1/2, Switch/1
  Sum1/1 -> Product2/1
  Relational Operator2/1 -> Logical Operator/1
  Relational Operator1/1 -> Logical Operator/2
  Logical Operator/1 -> Switch/2
  Memory1/1 -> Sum1/1, Relational Operator2/1, Switch/3
  PINLV_Hz/1 -> Gain1/1
  XIANGWEI_du/1 -> Math Function1/1
  Math Function1/1 -> Gain2/1
  mod/1 -> Math Function1/2
  bias_du/1 -> Sum2/2
  Sum2/1 -> sin_out/1
  Product3/1 -> Sum2/1

== system Copy_of_shake_table/Signal Generator/square_enable ==
  In1 : Inport  OutDataType=sfix(16)  OutScaling=2^0
  Enable : EnablePort  StatesWhenEnabling=reset
  Out1 : Outport  OutDataType=sfix(16)  OutScaling=2^0
  wires:
  In1/1 -> Out1/1

== system Copy_of_shake_table/tvc_filter/filter ==
  uxa : Inport  OutDataType=sfix(16)  OutScaling=2^0
  Dxf : Gain  Orientation=left  Gain=0.5*6.28*0.5*6.28  ParameterDataType=sfix(16)  ParameterScaling=2^0  OutDataType=sfix(16)  OutScaling=2^0  SaturateOnIntegerOverflow=on
  Integrator : Integrator
  Integrator1 : Integrator
  Sum : Sum  Inputs=+--  OutDataType=sfix(16)  OutScaling=2^0  SaturateOnIntegerOverflow=on
  Vxf : Gain  Orientation=left  Gain=2*0.7*0.5*6.28  ParameterDataType=sfix(16)  ParameterScaling=2^0  OutDataType=sfix(16)  OutScaling=2^0  SaturateOnIntegerOverflow=on
  ax : Outport  OutDataType=sfix(16)  OutScaling=2^0
  vx : Outport  Port=2  OutDataType=sfix(16)  OutScaling=2^0
  dx : Outport  Port=3  OutDataType=sfix(16)  OutScaling=2^0
  wires:
  Integrator1/1 -> Dxf/1, dx/1
  uxa/1 -> Sum/1
  Dxf/1 -> Sum/2
  Vxf/1 -> Sum/3
  Integrator/1 -> vx/1, Vxf/1, Integrator1/1
  Sum/1 -> ax/1, Integrator/1

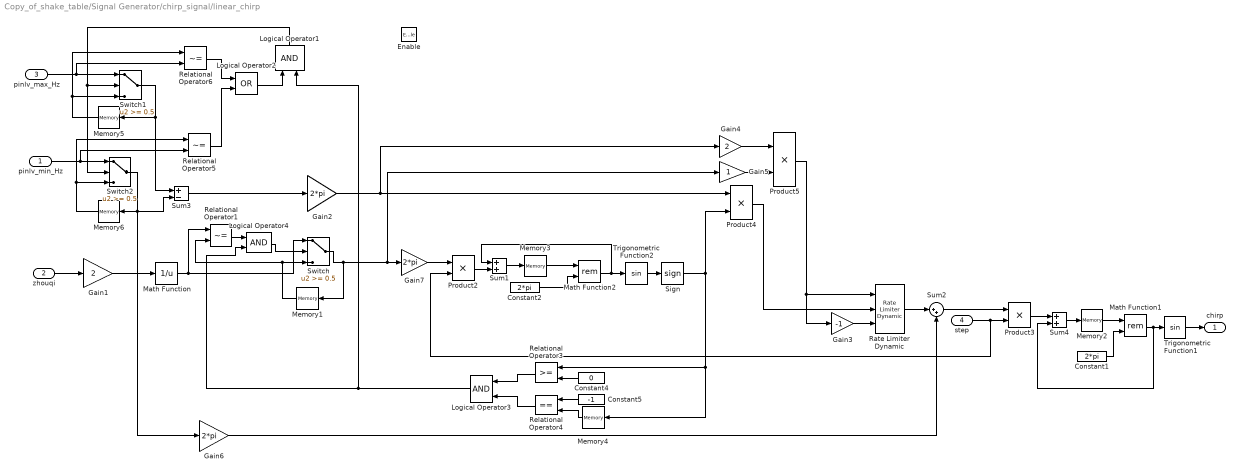
== system Copy_of_shake_table/Signal Generator/chirp_signal/linear_chirp ==
  pinlv_min_Hz : Inport  OutDataType=sfix(16)  OutScaling=2^0
  zhouqi : Inport  Port=2  OutDataType=sfix(16)  OutScaling=2^0
  pinlv_max_Hz : Inport  Port=3  OutDataType=sfix(16)  OutScaling=2^0
  step : Inport  Port=4  OutDataType=sfix(16)  OutScaling=2^0
  Enable : EnablePort  StatesWhenEnabling=reset
  Constant1 : Constant  Value=2*pi  OutDataType=sfix(16)  OutScaling=2^0
  Constant2 : Constant  Value=2*pi  OutDataType=sfix(16)  OutScaling=2^0
  Constant4 : Constant  Orientation=left  Value=0  OutDataType=sfix(16)  OutScaling=2^0
  Constant5 : Constant  Orientation=left  Value=-1  OutDataType=sfix(16)  OutScaling=2^0
  Gain1 : Gain  Gain=2  ParameterDataType=sfix(16)  ParameterScaling=2^0  OutDataType=sfix(16)  OutScaling=2^0  SaturateOnIntegerOverflow=on
  Gain2 : Gain  Gain=2*pi  ParameterDataType=sfix(16)  ParameterScaling=2^0  OutDataType=sfix(16)  OutScaling=2^0  SaturateOnIntegerOverflow=on
  Gain3 : Gain  Gain=-1  ParameterDataType=sfix(16)  ParameterScaling=2^0  OutDataType=sfix(16)  OutScaling=2^0  SaturateOnIntegerOverflow=on
  Gain4 : Gain  Gain=2  ParameterDataType=sfix(16)  ParameterScaling=2^0  OutDataType=sfix(16)  OutScaling=2^0  SaturateOnIntegerOverflow=on
  Gain5 : Gain  ParameterDataType=sfix(16)  ParameterScaling=2^0  OutDataType=sfix(16)  OutScaling=2^0  SaturateOnIntegerOverflow=on
  Gain6 : Gain  Gain=2*pi  ParameterDataType=sfix(16)  ParameterScaling=2^0  OutDataType=sfix(16)  OutScaling=2^0  SaturateOnIntegerOverflow=on
  Gain7 : Gain  Gain=2*pi  ParameterDataType=sfix(16)  ParameterScaling=2^0  OutDataType=sfix(16)  OutScaling=2^0  SaturateOnIntegerOverflow=on
  Logical Operator1 : Logic  Orientation=up  AllPortsSameDT=off
  Logical Operator2 : Logic  Operator=OR  AllPortsSameDT=off
  Logical Operator3 : Logic  Orientation=left  AllPortsSameDT=off
  Logical Operator4 : Logic  AllPortsSameDT=off
  Math Function : Math  Operator=reciprocal  OutDataType=sfix(16)  OutScaling=2^0  SaturateOnIntegerOverflow=on
  Math Function1 : Math  Operator=rem  OutDataType=sfix(16)  OutScaling=2^0  SaturateOnIntegerOverflow=on
  Math Function2 : Math  Operator=rem  OutDataType=sfix(16)  OutScaling=2^0  SaturateOnIntegerOverflow=on
  Memory1 : Memory  Orientation=left  X0=0.01
  Memory2 : Memory
  Memory3 : Memory  X0=2*pi-0.001
  Memory4 : Memory  Orientation=left
  Memory5 : Memory  Orientation=left
  Memory6 : Memory  Orientation=left
  Product{2..5} (4 alike) : Product  OutDataType=sfix(16)  OutScaling=2^0  SaturateOnIntegerOverflow=on
  Rate Limiter Dynamic : simulink/Discontinuities/Rate Limiter Dynamic  SystemSampleTime=-1
  Relational Operator1 : RelationalOperator  Operator=~=
  Relational Operator3 : RelationalOperator  Orientation=left
  Relational Operator4 : RelationalOperator  Orientation=left  Operator===
  Relational Operator5 : RelationalOperator  Operator=~=
  Relational Operator6 : RelationalOperator  Operator=~=
  Sign : Signum
  Sum1 : Sum  OutDataType=sfix(16)  OutScaling=2^0  SaturateOnIntegerOverflow=on
  Sum2 : Sum  Inputs=|++  OutDataType=sfix(16)  OutScaling=2^0  SaturateOnIntegerOverflow=on
  Sum3 : Sum  Inputs=+-  OutDataType=sfix(16)  OutScaling=2^0  SaturateOnIntegerOverflow=on
  Sum4 : Sum  OutDataType=sfix(16)  OutScaling=2^0  SaturateOnIntegerOverflow=on
  Switch : Switch  Threshold=0.5  SaturateOnIntegerOverflow=on
  Switch1 : Switch  Threshold=0.5  SaturateOnIntegerOverflow=on
  Switch2 : Switch  Threshold=0.5  SaturateOnIntegerOverflow=on
  Trigonometric Function1 : Trigonometry
  Trigonometric Function2 : Trigonometry
  chirp : Outport  OutDataType=sfix(16)  OutScaling=2^0
  wires:
  Gain2/1 -> Product4/1, Gain4/1
  Gain3/1 -> Rate Limiter Dynamic/3
  Gain4/1 -> Product5/1
  Gain5/1 -> Product5/2
  Product4/1 -> Rate Limiter Dynamic/2
  Product5/1 -> Gain3/1, Rate Limiter Dynamic/1
  zhouqi/1 -> Gain1/1
  Math Function/1 -> Relational Operator1/1, Switch/1
  Sum3/1 -> Gain2/1
  Rate Limiter Dynamic/1 -> Sum2/1
  Sum2/1 -> Product3/1
  Product3/1 -> Sum4/1
  step/1 -> Product3/2, Product2/2
  Sum4/1 -> Memory2/1
  Memory2/1 -> Math Function1/1
  Constant1/1 -> Math Function1/2
  Math Function1/1 -> Sum4/2, Trigonometric Function1/1
  Gain6/1 -> Sum2/2
  Switch/1 -> Memory1/1, Gain5/1, Gain7/1
  Memory1/1 -> Relational Operator1/2, Switch/3
  Trigonometric Function2/1 -> Sign/1
  Trigonometric Function1/1 -> chirp/1
  Memory4/1 -> Relational Operator4/2
  Constant5/1 -> Relational Operator4/1
  Switch1/1 -> Memory5/1, Sum3/1
  Memory5/1 -> Relational Operator6/1, Switch1/3
  pinlv_max_Hz/1 -> Relational Operator6/2, Switch1/1
  pinlv_min_Hz/1 -> Relational Operator5/2, Switch2/1
  Memory6/1 -> Relational Operator5/1, Switch2/3
  Switch2/1 -> Memory6/1, Sum3/2, Gain6/1
  Relational Operator6/1 -> Logical Operator2/1
  Relational Operator5/1 -> Logical Operator2/2
  Logical Operator2/1 -> Logical Operator1/1
  Logical Operator1/1 -> Switch1/2, Switch2/2
  Relational Operator3/1 -> Logical Operator3/1
  Relational Operator4/1 -> Logical Operator3/2
  Memory3/1 -> Math Function2/1
  Math Function2/1 -> Trigonometric Function2/1, Sum1/1
  Constant2/1 -> Math Function2/2
  Logical Operator3/1 -> Logical Operator4/2, Logical Operator1/2
  Sum1/1 -> Memory3/1
  Product2/1 -> Sum1/2
  Constant4/1 -> Relational Operator3/2
  Gain7/1 -> Product2/1
  Sign/1 -> Product4/2, Memory4/1, Relational Operator3/1
  Relational Operator1/1 -> Logical Operator4/1
  Logical Operator4/1 -> Switch/2
  Gain1/1 -> Math Function/1

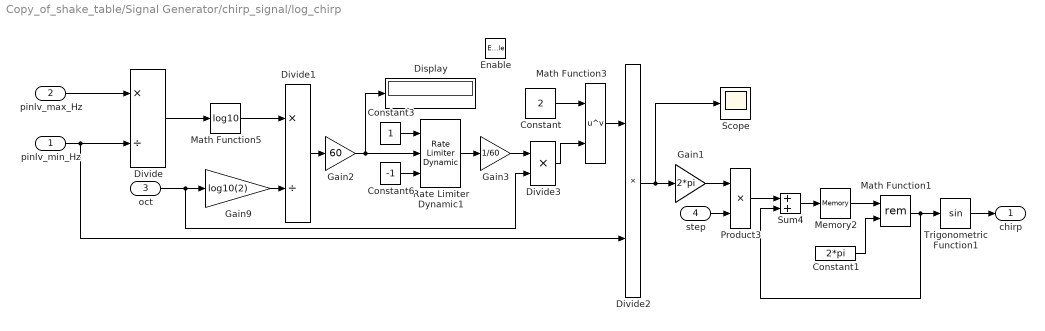
== system Copy_of_shake_table/Signal Generator/chirp_signal/log_chirp ==
  pinlv_min_Hz : Inport  OutDataType=sfix(16)  OutScaling=2^0
  pinlv_max_Hz : Inport  Port=2  OutDataType=sfix(16)  OutScaling=2^0
  oct : Inport  Port=3  OutDataType=sfix(16)  OutScaling=2^0
  step : Inport  Port=4  OutDataType=sfix(16)  OutScaling=2^0
  Enable : EnablePort  StatesWhenEnabling=reset
  Constant : Constant  Value=2  OutDataType=sfix(16)  OutScaling=2^0
  Constant1 : Constant  Value=2*pi  OutDataType=sfix(16)  OutScaling=2^0
  Constant3 : Constant  OutDataType=sfix(16)  OutScaling=2^0
  Constant6 : Constant  Value=-1  OutDataType=sfix(16)  OutScaling=2^0
  Display : Display
  Divide : Product  Inputs=*/  OutDataTypeMode=double  OutDataType=sfix(16)  OutScaling=2^-10
  Divide1 : Product  Inputs=*/  OutDataTypeMode=double  OutDataType=sfix(16)  OutScaling=2^-10
  Divide2 : Product  Inputs=**  OutDataTypeMode=double  OutDataType=sfix(16)  OutScaling=2^-10
  Divide3 : Product  Inputs=**  OutDataTypeMode=double  OutDataType=sfix(16)  OutScaling=2^-10
  Gain1 : Gain  Gain=2*pi  ParameterDataType=sfix(16)  ParameterScaling=2^0  OutDataType=sfix(16)  OutScaling=2^0  SaturateOnIntegerOverflow=on
  Gain2 : Gain  Gain=60  ParameterDataType=sfix(16)  ParameterScaling=2^0  OutDataType=sfix(16)  OutScaling=2^0  SaturateOnIntegerOverflow=on
  Gain3 : Gain  Gain=1/60  ParameterDataType=sfix(16)  ParameterScaling=2^0  OutDataType=sfix(16)  OutScaling=2^0  SaturateOnIntegerOverflow=on
  Gain9 : Gain  Gain=log10(2)  ParameterDataType=sfix(16)  ParameterScaling=2^0  OutDataType=sfix(16)  OutScaling=2^0  SaturateOnIntegerOverflow=on
  Math Function1 : Math  Operator=rem  OutDataType=sfix(16)  OutScaling=2^0  SaturateOnIntegerOverflow=on
  Math Function3 : Math  Operator=pow  OutDataType=sfix(16)  OutScaling=2^0  SaturateOnIntegerOverflow=on
  Math Function5 : Math  Operator=log10  OutDataType=sfix(16)  OutScaling=2^0  SaturateOnIntegerOverflow=on
  Memory2 : Memory
  Product3 : Product  OutDataType=sfix(16)  OutScaling=2^0  SaturateOnIntegerOverflow=on
  Rate Limiter Dynamic1 : simulink/Discontinuities/Rate Limiter Dynamic  SystemSampleTime=-1
  Scope : Scope
      settings: SaveName=ScopeData5
  Sum4 : Sum  OutDataType=sfix(16)  OutScaling=2^0  SaturateOnIntegerOverflow=on
  Trigonometric Function1 : Trigonometry
  chirp : Outport  OutDataType=sfix(16)  OutScaling=2^0
  wires:
  Constant6/1 -> Rate Limiter Dynamic1/3
  Constant3/1 -> Rate Limiter Dynamic1/1
  Gain3/1 -> Divide3/1
  Gain1/1 -> Product3/1
  Product3/1 -> Sum4/1
  step/1 -> Product3/2
  Sum4/1 -> Memory2/1
  Memory2/1 -> Math Function1/1
  Constant1/1 -> Math Function1/2
  Math Function1/1 -> Trigonometric Function1/1, Sum4/2
  Rate Limiter Dynamic1/1 -> Gain3/1
  Gain2/1 -> Display/1, Rate Limiter Dynamic1/2
  Divide2/1 -> Scope/1, Gain1/1
  Math Function3/1 -> Divide2/1
  Trigonometric Function1/1 -> chirp/1
  Divide3/1 -> Math Function3/2
  Constant/1 -> Math Function3/1
  Divide1/1 -> Gain2/1
  Gain9/1 -> Divide1/2
  Math Function5/1 -> Divide1/1
  oct/1 -> Divide3/2, Gain9/1
  Divide/1 -> Math Function5/1
  pinlv_min_Hz/1 -> Divide2/2, Divide/2
  pinlv_max_Hz/1 -> Divide/1

== stateflow chart Nomal Motion Logic/Control Logic ==
  state run_mode [parallel]
    settings: executionOrder=1
    state running
      du:start=1;start_sts=2;
    state to_stopped
      du:start=0;start_sts=3;
    state to_running
      du:start=1;start_sts=1;
    state stopped
      du:start=0;start_sts=0;
    (default) -> stopped
    stopped -> to_running : [start_cmd&&in(ready_mode.ready)]
    to_running -> running [order 1] : [start_cmd==start_fbk]
    running -> to_stopped : [!start_cmd]
    to_stopped -> stopped [order 2] : [start_cmd==start_fbk]
    to_stopped -> to_running [order 1] : [start_cmd&&in(ready_mode.ready)]
    to_running -> to_stopped [order 2] : [!start_cmd]
  state ready_mode [parallel]
    settings: executionOrder=2
    state ready
      du:ready=1;ready_sts=2;
    state to_rest
      du:ready=0;ready_sts=3;
    state rest
      du:ready=0;ready_sts=0;
    state to_ready
      du:ready=1;ready_sts=1;
    (default) -> rest
    rest -> to_ready : [ready_cmd]
    to_ready -> ready [order 1] : [ready_cmd==ready_fbk]
    ready -> to_rest : [!ready_cmd&&in(run_mode.stopped)]
    to_rest -> rest [order 2] : [ready_cmd==ready_fbk]
    to_rest -> to_ready [order 1] : [ready_cmd]
    to_ready -> to_rest [order 2] : [!ready_cmd&&in(run_mode.stopped)]
  data: start_fbk input double; start_cmd input double; ready_cmd input double; ready_fbk input double; start output boolean; start_sts output double; ready_sts output double; ready output boolean
